simulink model "multilevel_inverter"  (R2021b)
settings: Solver=ode45  StartTime=0.0  StopTime=0.1  RelTol=1e-3  EnableMultiTasking=on
libraries: spsIGBTLib x32, spsDCVoltageSourceLib x8, spsVoltageMeasurementLib x1, spspowerguiLib x1
settings Model: Creator=amit  LastModifiedBy=HP
settings SolverCC: AlgebraicLoopSolver=TrustRegion
settings DataIOCC: LimitDataPoints=on  SaveFormat=Array  SignalLoggingSaveFormat=ModelDataLogs  ReturnWorkspaceOutputs=off
settings OptimizationCC: ExpressionDepthLimit=2147483647  LifeSpan=inf
settings DebuggingCC: UnderspecifiedInitializationDetection=Classic  MergeDetectMultiDrivingBlocksExec=none  FcnCallInpInsideContextMsg=warning  StateNameClashWarn=warning  SFUnexpectedBacktrackingDiag=warning  SFNoUnconditionalDefaultTransitionDiag=warning  SFExecutionAtInitializationDiag=none  SFMachineParentedDataDiag=warning  ArithmeticOperatorsInVariantConditions=warning
settings HardwareCC: ProdBitPerPointer=32  ProdBitPerSizeT=32  ProdBitPerPtrDiffT=32  ProdLargestAtomicFloat=None  ProdIntDivRoundTo=Undefined  ProdEndianess=Unspecified  ProdWordSize=32  ProdHWDeviceType=32-bit Generic
settings ModelReferenceCC: PropagateSignalLabelsOutOfModel=off
settings SFSimCC: SimUseLocalCustomCode=off  CustomCodeUndefinedFunction=UseInterfaceOnly
settings RTWCC: RTWUseLocalCustomCode=off
settings CodeAppCC: StateflowObjectComments=on
settings GRTTargetCC: TargetLangStandard=C89/C90 (ANSI)  CombineOutputUpdateFcns=off  GRTInterface=on
settings ConfigComp: CovMetricSettings=dw  CovSaveCumulativeToWorkspaceVar=on  CovSaveSingleToWorkspaceVar=on  CovExternalEMLEnable=off

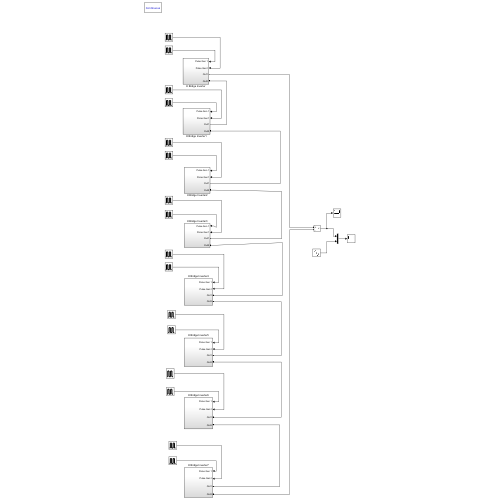
[thumbnail: Simulink's stored preview of the top-level diagram]
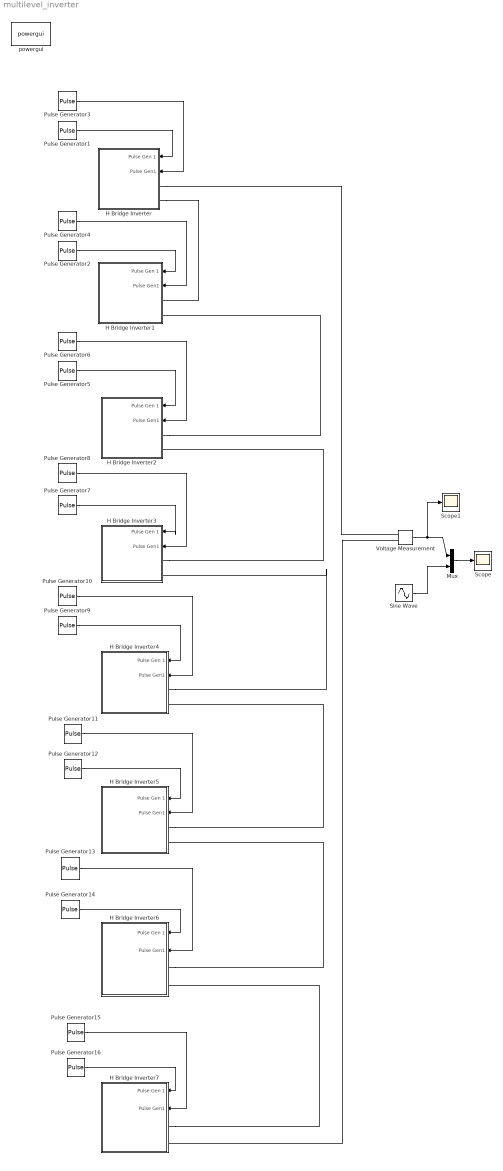
== system multilevel_inverter ==
  H Bridge Inverter : Subsystem
  H Bridge Inverter1 : Subsystem
  H Bridge Inverter2 : Subsystem
  H Bridge Inverter3 : Subsystem
  H Bridge Inverter4 : Subsystem
  H Bridge Inverter5 : Subsystem
  H Bridge Inverter6 : Subsystem
  H Bridge Inverter7 : Subsystem
  Mux : Mux  Inputs=2
  Pulse Generator1 : DiscretePulseGenerator  PulseType=Time based  Period=0.02  PulseWidth=45  PhaseDelay=0.0005
  Pulse Generator10 : DiscretePulseGenerator  PulseType=Time based  Period=0.02  PulseWidth=25  PhaseDelay=0.0125
  Pulse Generator11 : DiscretePulseGenerator  PulseType=Time based  Period=0.02  PulseWidth=20  PhaseDelay=0.0130
  Pulse Generator12 : DiscretePulseGenerator  PulseType=Time based  Period=0.02  PulseWidth=20  PhaseDelay=0.0030
  Pulse Generator13 : DiscretePulseGenerator  PulseType=Time based  Period=0.02  PulseWidth=15  PhaseDelay=0.0135
  Pulse Generator14 : DiscretePulseGenerator  PulseType=Time based  Period=0.02  PulseWidth=15  PhaseDelay=0.0035
  Pulse Generator15 : DiscretePulseGenerator  PulseType=Time based  Period=0.02  PulseWidth=10  PhaseDelay=0.0140
  Pulse Generator16 : DiscretePulseGenerator  PulseType=Time based  Period=0.02  PulseWidth=10  PhaseDelay=0.0040
  Pulse Generator2 : DiscretePulseGenerator  PulseType=Time based  Period=0.02  PulseWidth=40  PhaseDelay=0.001
  Pulse Generator3 : DiscretePulseGenerator  PulseType=Time based  Period=0.02  PulseWidth=45  PhaseDelay=0.0105
  Pulse Generator4 : DiscretePulseGenerator  PulseType=Time based  Period=0.02  PulseWidth=40  PhaseDelay=0.011
  Pulse Generator5 : DiscretePulseGenerator  PulseType=Time based  Period=0.02  PulseWidth=35  PhaseDelay=0.0015
  Pulse Generator6 : DiscretePulseGenerator  PulseType=Time based  Period=0.02  PulseWidth=35  PhaseDelay=0.0115
  Pulse Generator7 : DiscretePulseGenerator  PulseType=Time based  Period=0.02  PulseWidth=30  PhaseDelay=0.0020
  Pulse Generator8 : DiscretePulseGenerator  PulseType=Time based  Period=0.02  PulseWidth=30  PhaseDelay=0.0120
  Pulse Generator9 : DiscretePulseGenerator  PulseType=Time based  Period=0.02  PulseWidth=25  PhaseDelay=0.0025
  Scope : Scope
  Scope1 : Scope
  Sine Wave : Sin  Amplitude=8  Frequency=314  SampleTime=0
  Voltage Measurement : spsVoltageMeasurementLib/Voltage Measurement  PhasorSimulation=off  OutputType=Complex  PSBequivalent=0
  powergui : spspowerguiLib/powergui  Priority=1  SimulationMode=Continuous  SampleTime=50e-6  frequency=60  Iterations=50  frequencyindice=0  Pbase=100e6  ErrMax=1e-4  UnitsV=kV  UnitsW=MW  buscounter=0  FunctionMessages=on  echomessages=off  EnableUseOfTLC=off  CurrentSourceSwitches=on  DisableSnubberDevices=off  DisableRonSwitches=off  DisableVfSwitches=off  DisplayEquations=off  AutomaticDiscreteSolvers=off  SolverType=Tustin/Backward Euler (TBE)  Interpol=off  ExternalGateDelay=off  methode=off  Ts=0  x0status=blocks  SPID=off  SwTol=0  HookPort=off  NonlinearTolerance=1e-4  nMaxIteration=100  ContinueOnMaxIteration=off  RestoreLinks=warning  ResistiveCurrentMeasurement=off  Frange=[0:2:500]  Ylog=off  Xlog=on  ShowGrid=off  save=off  variable=ZData  structure=0  ZoomFFT=on  StartTime=0.0  cycles=1  DisplayStyle=1  fundamental=60  FreqAxis=off  MaxFrequency=1000  frequencyindicesteady=1  RmsSteady=1  display=off
  wires:
  Pulse Generator1/1 -> H Bridge Inverter/1(Pulse Gen 1)
  Pulse Generator3/1 -> H Bridge Inverter/2(Pulse Gen1)
  Pulse Generator2/1 -> H Bridge Inverter1/1(Pulse Gen 1)
  Pulse Generator4/1 -> H Bridge Inverter1/2(Pulse Gen1)
  Pulse Generator5/1 -> H Bridge Inverter2/1(Pulse Gen 1)
  Pulse Generator6/1 -> H Bridge Inverter2/2(Pulse Gen1)
  Pulse Generator7/1 -> H Bridge Inverter3/1(Pulse Gen 1)
  Pulse Generator8/1 -> H Bridge Inverter3/2(Pulse Gen1)
  Sine Wave/1 -> Mux/2
  Voltage Measurement/1 -> Mux/1, Scope1/1
  Mux/1 -> Scope/1
  Pulse Generator9/1 -> H Bridge Inverter4/1(Pulse Gen 1)
  Pulse Generator10/1 -> H Bridge Inverter4/2(Pulse Gen1)
  Pulse Generator12/1 -> H Bridge Inverter5/1(Pulse Gen 1)
  Pulse Generator11/1 -> H Bridge Inverter5/2(Pulse Gen1)
  Pulse Generator14/1 -> H Bridge Inverter6/1(Pulse Gen 1)
  Pulse Generator13/1 -> H Bridge Inverter6/2(Pulse Gen1)
  Pulse Generator16/1 -> H Bridge Inverter7/1(Pulse Gen 1)
  Pulse Generator15/1 -> H Bridge Inverter7/2(Pulse Gen1)
  connections:
  H Bridge Inverter/LConn1 -- Voltage Measurement/LConn1
  H Bridge Inverter/LConn2 -- H Bridge Inverter1/LConn1
  H Bridge Inverter2/LConn1 -- H Bridge Inverter1/LConn2
  H Bridge Inverter3/LConn1 -- H Bridge Inverter2/LConn2
  H Bridge Inverter4/LConn1 -- H Bridge Inverter3/LConn2
  H Bridge Inverter5/LConn1 -- H Bridge Inverter4/LConn2
  H Bridge Inverter6/LConn1 -- H Bridge Inverter5/LConn2
  H Bridge Inverter7/LConn1 -- H Bridge Inverter6/LConn2
  Voltage Measurement/LConn2 -- H Bridge Inverter7/LConn2

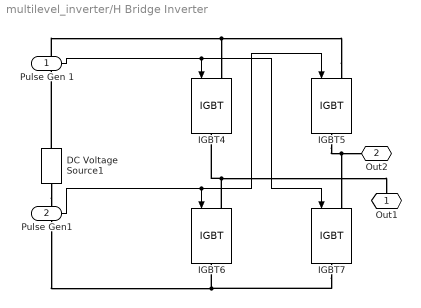
== system multilevel_inverter/H Bridge Inverter ==
  Pulse Gen 1 : Inport
  Pulse Gen1 : Inport  Port=2
  DC Voltage Source1 : spsDCVoltageSourceLib/DC Voltage Source  Amplitude=3  Measurements=None
  IGBT{4..7} (4 alike) : spsIGBTLib/IGBT  Ron=0.001  Lon=0  Vf=1  Tf=1e-6  Tt=2e-6  IC=0  Rs=1e5  Cs=inf  Measurements=off
  Out1 : PMIOPort  Side=Left
  Out2 : PMIOPort  Port=2  Side=Left
  wires:
  Pulse Gen 1/1 -> IGBT7/1, IGBT4/1
  Pulse Gen1/1 -> IGBT5/1, IGBT6/1
  connections:
  IGBT7/RConn1 -- DC Voltage Source1/LConn1 -- IGBT6/RConn1
  IGBT5/LConn1 -- DC Voltage Source1/RConn1 -- IGBT4/LConn1
  Out1/RConn1 -- IGBT4/RConn1 -- IGBT6/LConn1
  IGBT5/RConn1 -- Out2/RConn1 -- IGBT7/LConn1

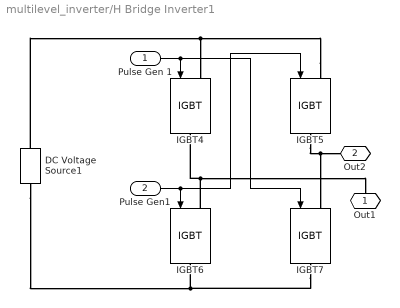
== system multilevel_inverter/H Bridge Inverter1 ==
  Pulse Gen 1 : Inport
  Pulse Gen1 : Inport  Port=2
  DC Voltage Source1 : spsDCVoltageSourceLib/DC Voltage Source  Amplitude=3  Measurements=None
  IGBT{4..7} (4 alike) : spsIGBTLib/IGBT  Ron=0.001  Lon=0  Vf=1  Tf=1e-6  Tt=2e-6  IC=0  Rs=1e5  Cs=inf  Measurements=off
  Out1 : PMIOPort  Side=Left
  Out2 : PMIOPort  Port=2  Side=Left
  wires:
  Pulse Gen 1/1 -> IGBT7/1, IGBT4/1
  Pulse Gen1/1 -> IGBT5/1, IGBT6/1
  connections:
  IGBT7/RConn1 -- DC Voltage Source1/LConn1 -- IGBT6/RConn1
  IGBT5/LConn1 -- DC Voltage Source1/RConn1 -- IGBT4/LConn1
  Out1/RConn1 -- IGBT4/RConn1 -- IGBT6/LConn1
  IGBT5/RConn1 -- Out2/RConn1 -- IGBT7/LConn1

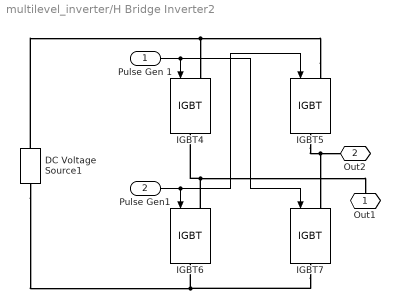
== system multilevel_inverter/H Bridge Inverter2 ==
  Pulse Gen 1 : Inport
  Pulse Gen1 : Inport  Port=2
  DC Voltage Source1 : spsDCVoltageSourceLib/DC Voltage Source  Amplitude=3  Measurements=None
  IGBT{4..7} (4 alike) : spsIGBTLib/IGBT  Ron=0.001  Lon=0  Vf=1  Tf=1e-6  Tt=2e-6  IC=0  Rs=1e5  Cs=inf  Measurements=off
  Out1 : PMIOPort  Side=Left
  Out2 : PMIOPort  Port=2  Side=Left
  wires:
  Pulse Gen 1/1 -> IGBT7/1, IGBT4/1
  Pulse Gen1/1 -> IGBT5/1, IGBT6/1
  connections:
  IGBT7/RConn1 -- DC Voltage Source1/LConn1 -- IGBT6/RConn1
  IGBT5/LConn1 -- DC Voltage Source1/RConn1 -- IGBT4/LConn1
  Out1/RConn1 -- IGBT4/RConn1 -- IGBT6/LConn1
  IGBT5/RConn1 -- Out2/RConn1 -- IGBT7/LConn1

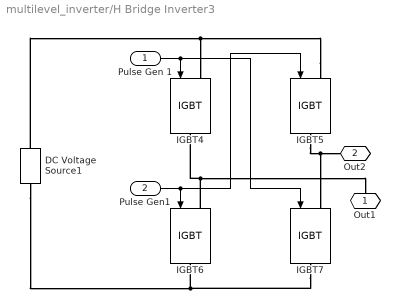
== system multilevel_inverter/H Bridge Inverter3 ==
  Pulse Gen 1 : Inport
  Pulse Gen1 : Inport  Port=2
  DC Voltage Source1 : spsDCVoltageSourceLib/DC Voltage Source  Amplitude=3  Measurements=None
  IGBT{4..7} (4 alike) : spsIGBTLib/IGBT  Ron=0.001  Lon=0  Vf=1  Tf=1e-6  Tt=2e-6  IC=0  Rs=1e5  Cs=inf  Measurements=off
  Out1 : PMIOPort  Side=Left
  Out2 : PMIOPort  Port=2  Side=Left
  wires:
  Pulse Gen 1/1 -> IGBT7/1, IGBT4/1
  Pulse Gen1/1 -> IGBT5/1, IGBT6/1
  connections:
  IGBT7/RConn1 -- DC Voltage Source1/LConn1 -- IGBT6/RConn1
  IGBT5/LConn1 -- DC Voltage Source1/RConn1 -- IGBT4/LConn1
  Out1/RConn1 -- IGBT4/RConn1 -- IGBT6/LConn1
  IGBT5/RConn1 -- Out2/RConn1 -- IGBT7/LConn1

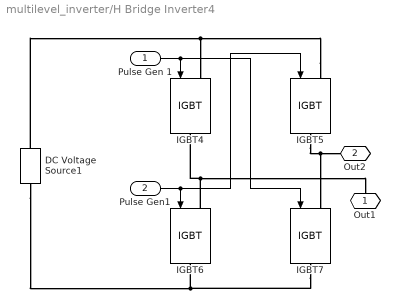
== system multilevel_inverter/H Bridge Inverter4 ==
  Pulse Gen 1 : Inport
  Pulse Gen1 : Inport  Port=2
  DC Voltage Source1 : spsDCVoltageSourceLib/DC Voltage Source  Amplitude=3  Measurements=None
  IGBT{4..7} (4 alike) : spsIGBTLib/IGBT  Ron=0.001  Lon=0  Vf=1  Tf=1e-6  Tt=2e-6  IC=0  Rs=1e5  Cs=inf  Measurements=off
  Out1 : PMIOPort  Side=Left
  Out2 : PMIOPort  Port=2  Side=Left
  wires:
  Pulse Gen 1/1 -> IGBT7/1, IGBT4/1
  Pulse Gen1/1 -> IGBT5/1, IGBT6/1
  connections:
  IGBT7/RConn1 -- DC Voltage Source1/LConn1 -- IGBT6/RConn1
  IGBT5/LConn1 -- DC Voltage Source1/RConn1 -- IGBT4/LConn1
  Out1/RConn1 -- IGBT4/RConn1 -- IGBT6/LConn1
  IGBT5/RConn1 -- Out2/RConn1 -- IGBT7/LConn1

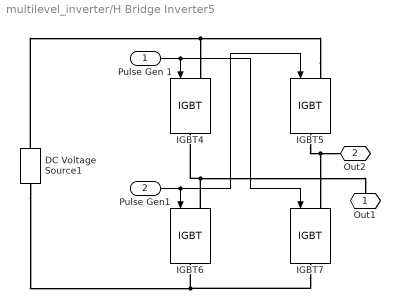
== system multilevel_inverter/H Bridge Inverter5 ==
  Pulse Gen 1 : Inport
  Pulse Gen1 : Inport  Port=2
  DC Voltage Source1 : spsDCVoltageSourceLib/DC Voltage Source  Amplitude=3  Measurements=None
  IGBT{4..7} (4 alike) : spsIGBTLib/IGBT  Ron=0.001  Lon=0  Vf=1  Tf=1e-6  Tt=2e-6  IC=0  Rs=1e5  Cs=inf  Measurements=off
  Out1 : PMIOPort  Side=Left
  Out2 : PMIOPort  Port=2  Side=Left
  wires:
  Pulse Gen 1/1 -> IGBT7/1, IGBT4/1
  Pulse Gen1/1 -> IGBT5/1, IGBT6/1
  connections:
  IGBT7/RConn1 -- DC Voltage Source1/LConn1 -- IGBT6/RConn1
  IGBT5/LConn1 -- DC Voltage Source1/RConn1 -- IGBT4/LConn1
  Out1/RConn1 -- IGBT4/RConn1 -- IGBT6/LConn1
  IGBT5/RConn1 -- Out2/RConn1 -- IGBT7/LConn1

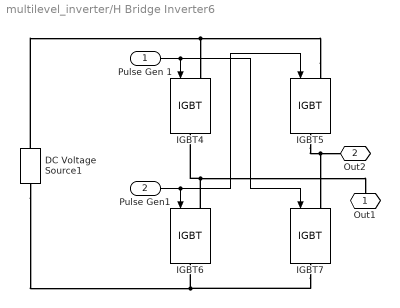
== system multilevel_inverter/H Bridge Inverter6 ==
  Pulse Gen 1 : Inport
  Pulse Gen1 : Inport  Port=2
  DC Voltage Source1 : spsDCVoltageSourceLib/DC Voltage Source  Amplitude=3  Measurements=None
  IGBT{4..7} (4 alike) : spsIGBTLib/IGBT  Ron=0.001  Lon=0  Vf=1  Tf=1e-6  Tt=2e-6  IC=0  Rs=1e5  Cs=inf  Measurements=off
  Out1 : PMIOPort  Side=Left
  Out2 : PMIOPort  Port=2  Side=Left
  wires:
  Pulse Gen 1/1 -> IGBT7/1, IGBT4/1
  Pulse Gen1/1 -> IGBT5/1, IGBT6/1
  connections:
  IGBT7/RConn1 -- DC Voltage Source1/LConn1 -- IGBT6/RConn1
  IGBT5/LConn1 -- DC Voltage Source1/RConn1 -- IGBT4/LConn1
  Out1/RConn1 -- IGBT4/RConn1 -- IGBT6/LConn1
  IGBT5/RConn1 -- Out2/RConn1 -- IGBT7/LConn1

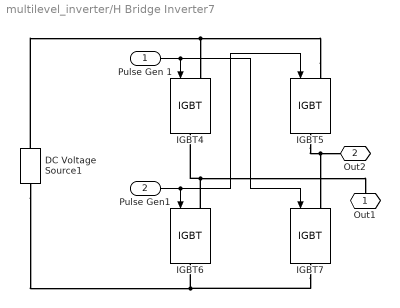
== system multilevel_inverter/H Bridge Inverter7 ==
  Pulse Gen 1 : Inport
  Pulse Gen1 : Inport  Port=2
  DC Voltage Source1 : spsDCVoltageSourceLib/DC Voltage Source  Amplitude=3  Measurements=None
  IGBT{4..7} (4 alike) : spsIGBTLib/IGBT  Ron=0.001  Lon=0  Vf=1  Tf=1e-6  Tt=2e-6  IC=0  Rs=1e5  Cs=inf  Measurements=off
  Out1 : PMIOPort  Side=Left
  Out2 : PMIOPort  Port=2  Side=Left
  wires:
  Pulse Gen 1/1 -> IGBT7/1, IGBT4/1
  Pulse Gen1/1 -> IGBT5/1, IGBT6/1
  connections:
  IGBT7/RConn1 -- DC Voltage Source1/LConn1 -- IGBT6/RConn1
  IGBT5/LConn1 -- DC Voltage Source1/RConn1 -- IGBT4/LConn1
  Out1/RConn1 -- IGBT4/RConn1 -- IGBT6/LConn1
  IGBT5/RConn1 -- Out2/RConn1 -- IGBT7/LConn1
